simulink model "atv4"  (R2018b)
settings: Solver=VariableStepAuto  StartTime=0.0  StopTime=10  RelTol=1e-3
settings Model: Creator=andre  LastModifiedBy=andre
settings DataIOCC: ReturnWorkspaceOutputs=on

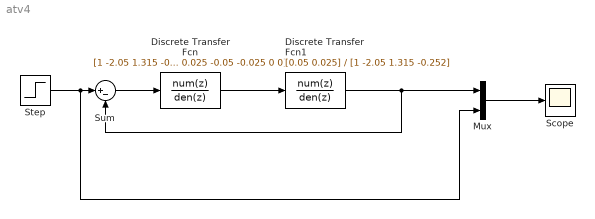
== system atv4 ==
  Discrete Transfer Fcn : DiscreteTransferFcn  Numerator=[1 -2.05 1.315 -0.252 0 0]  Denominator=[0.05 0.025 -0.05 -0.025 0 0]
  Discrete Transfer Fcn1 : DiscreteTransferFcn  Numerator=[0.05 0.025]  Denominator=[1 -2.05 1.315 -0.252]
  Mux : Mux  Inputs=2
  Scope : Scope
  Step : Step  SampleTime=0
  Sum : Sum  Inputs=|+-
  wires:
  Step/1 -> Mux/2, Sum/1
  Mux/1 -> Scope/1
  Discrete Transfer Fcn1/1 -> Sum/2, Mux/1
  Discrete Transfer Fcn/1 -> Discrete Transfer Fcn1/1
  Sum/1 -> Discrete Transfer Fcn/1
